simulink library "AEMS_Standard_Library"  (R2016b)
settings: Solver=ode45  StartTime=0.0  StopTime=10.0  RelTol=1e-3
undefined symbols (not defined in the file or in its folder): BkPY, carto, Cbx_extegr, Cbx_lpegrsys, Cbx_portegr, Cnx_bnk_nr_conf, Cnx_cyl_nr_conf, ConfigManagement, configuration_management, Cxx_dcm_io_tmr_end_xxxx, Cxx_dcm_rt_tmr_end, Cxx_DID_xxxx_IO_max, Cxx_DID_xxxx_IO_min, Cxx_egrhsofs, Cxx_vmaniegi, DEM_DEBOUNCE_FREEZE, DEM_DTR_CTL_INVISIBLE, DEM_DTR_CTL_NORMAL, Dem_DtrId2_XXX, Dem_DtrId3_XXX, Dem_DtrId4_XXX, Dem_DtrId5_XXX, Dem_DtrId6_XXX, Dem_DtrId7_XXX, Dem_DtrId8_XXX, Dem_DtrId9_XXX, Dem_DtrId_XXX, Dem_EnableConditionId2_XXX, Dem_EnableConditionId3_XXX, Dem_EnableConditionId4_XXX, Dem_EnableConditionId5_XXX, Dem_EnableConditionId6_XXX, Dem_EnableConditionId7_XXX, Dem_EnableConditionId8_XXX, Dem_EnableConditionId_XXX, Dem_EventId, Dem_EventId2_XXX, Dem_EventId3_XXX, Dem_EventId4_XXX, Dem_EventId5_XXX, Dem_EventId6_XXX, Dem_EventId7_XXX, Dem_EventId8_XXX, Dem_EventId9_XXX, Dem_EventId_Device_Faulttype, Dem_EventId_XXX, DEM_IUMPR_GENERAL_DENOMINATOR, DEM_OPCYC_IGNITION, Dem_RatioId2_XXX, Dem_RatioId3_XXX, Dem_RatioId4_XXX, Dem_RatioId5_XXX, Dem_RatioId6_XXX, Dem_RatioId7_XXX, Dem_RatioId8_XXX, Dem_RatioId_XXX, Dem_StorageConditionId2_XXX, Dem_StorageConditionId3_XXX, Dem_StorageConditionId4_XXX, Dem_StorageConditionId5_XXX ... (+65)
libraries: AEMS_Standard_Library x477, simulink x2
(part 34 of 39)

== system AEMS_Standard_Library/SUB/AEMS_DEM_SET_EVENT_STS_2D/Dem_SetEventStatus_Call2 ==
  dem_event_status_failed2 : Inport
  trigger_job_1st2 : EnablePort
      settings: AttributesFormatString=<states=%<StatesWhenEnabling>>
  AEMS_DEM_SETEVENTSTATUS2 : AEMS_Standard_Library/SUB/AEMS_DEM_SETEVENTSTATUS  Tag=[LIB]
      settings: AttributesFormatString=%<MaskType>
  EventId_block2 : Constant  Value=Dem_EventId2_XXX  OutDataTypeStr=uint16
  wires:
  EventId_block2/1 -> AEMS_DEM_SETEVENTSTATUS2/1
  dem_event_status_failed2/1 -> AEMS_DEM_SETEVENTSTATUS2/2

== system AEMS_Standard_Library/SUB/AEMS_DEM_SET_EVENT_STS_8D/Dem_SetEventStatus_Call1 ==
  dem_event_status_failed1 : Inport
  trigger_job_1st1 : EnablePort
      settings: AttributesFormatString=<states=%<StatesWhenEnabling>>
  AEMS_DEM_SETEVENTSTATUS1 : AEMS_Standard_Library/SUB/AEMS_DEM_SETEVENTSTATUS  Tag=[LIB]
      settings: AttributesFormatString=%<MaskType>
  EventId_block1 : Constant  Value=Dem_EventId_XXX  OutDataTypeStr=uint16
  wires:
  EventId_block1/1 -> AEMS_DEM_SETEVENTSTATUS1/1
  dem_event_status_failed1/1 -> AEMS_DEM_SETEVENTSTATUS1/2

== system AEMS_Standard_Library/SUB/AEMS_DEM_SET_EVENT_STS_8D/Dem_SetEventStatus_Call2 ==
  dem_event_status_failed2 : Inport
  trigger_job_1st2 : EnablePort
      settings: AttributesFormatString=<states=%<StatesWhenEnabling>>
  AEMS_DEM_SETEVENTSTATUS2 : AEMS_Standard_Library/SUB/AEMS_DEM_SETEVENTSTATUS  Tag=[LIB]
      settings: AttributesFormatString=%<MaskType>
  EventId_block2 : Constant  Value=Dem_EventId2_XXX  OutDataTypeStr=uint16
  wires:
  dem_event_status_failed2/1 -> AEMS_DEM_SETEVENTSTATUS2/2
  EventId_block2/1 -> AEMS_DEM_SETEVENTSTATUS2/1

== system AEMS_Standard_Library/SUB/AEMS_DEM_SET_EVENT_STS_8D/Dem_SetEventStatus_Call3 ==
  dem_event_status_failed3 : Inport
  trigger_job_1st3 : EnablePort
      settings: AttributesFormatString=<states=%<StatesWhenEnabling>>
  AEMS_DEM_SETEVENTSTATUS3 : AEMS_Standard_Library/SUB/AEMS_DEM_SETEVENTSTATUS  Tag=[LIB]
      settings: AttributesFormatString=%<MaskType>
  EventId_block3 : Constant  Value=Dem_EventId3_XXX  OutDataTypeStr=uint16
  wires:
  EventId_block3/1 -> AEMS_DEM_SETEVENTSTATUS3/1
  dem_event_status_failed3/1 -> AEMS_DEM_SETEVENTSTATUS3/2

== system AEMS_Standard_Library/SUB/AEMS_DEM_SET_EVENT_STS_8D/Dem_SetEventStatus_Call4 ==
  dem_event_status_failed4 : Inport
  trigger_job_1st4 : EnablePort
      settings: AttributesFormatString=<states=%<StatesWhenEnabling>>
  AEMS_DEM_SETEVENTSTATUS4 : AEMS_Standard_Library/SUB/AEMS_DEM_SETEVENTSTATUS  Tag=[LIB]
      settings: AttributesFormatString=%<MaskType>
  EventId_block4 : Constant  Value=Dem_EventId4_XXX  OutDataTypeStr=uint16
  wires:
  EventId_block4/1 -> AEMS_DEM_SETEVENTSTATUS4/1
  dem_event_status_failed4/1 -> AEMS_DEM_SETEVENTSTATUS4/2

== system AEMS_Standard_Library/SUB/AEMS_DEM_SET_EVENT_STS_8D/Dem_SetEventStatus_Call5 ==
  dem_event_status_failed5 : Inport
  trigger_job_1st5 : EnablePort
      settings: AttributesFormatString=<states=%<StatesWhenEnabling>>
  AEMS_DEM_SETEVENTSTATUS5 : AEMS_Standard_Library/SUB/AEMS_DEM_SETEVENTSTATUS  Tag=[LIB]
      settings: AttributesFormatString=%<MaskType>
  EventId_block5 : Constant  Value=Dem_EventId5_XXX  OutDataTypeStr=uint16
  wires:
  dem_event_status_failed5/1 -> AEMS_DEM_SETEVENTSTATUS5/2
  EventId_block5/1 -> AEMS_DEM_SETEVENTSTATUS5/1

== system AEMS_Standard_Library/SUB/AEMS_DEM_SET_EVENT_STS_8D/Dem_SetEventStatus_Call6 ==
  dem_event_status_failed6 : Inport
  trigger_job_1st6 : EnablePort
      settings: AttributesFormatString=<states=%<StatesWhenEnabling>>
  AEMS_DEM_SETEVENTSTATUS6 : AEMS_Standard_Library/SUB/AEMS_DEM_SETEVENTSTATUS  Tag=[LIB]
      settings: AttributesFormatString=%<MaskType>
  EventId_block6 : Constant  Value=Dem_EventId6_XXX  OutDataTypeStr=uint16
  wires:
  EventId_block6/1 -> AEMS_DEM_SETEVENTSTATUS6/1
  dem_event_status_failed6/1 -> AEMS_DEM_SETEVENTSTATUS6/2

== system AEMS_Standard_Library/SUB/AEMS_DEM_SET_EVENT_STS_8D/Dem_SetEventStatus_Call7 ==
  dem_event_status_failed7 : Inport
  trigger_job_1st7 : EnablePort
      settings: AttributesFormatString=<states=%<StatesWhenEnabling>>
  AEMS_DEM_SETEVENTSTATUS7 : AEMS_Standard_Library/SUB/AEMS_DEM_SETEVENTSTATUS  Tag=[LIB]
      settings: AttributesFormatString=%<MaskType>
  EventId_block7 : Constant  Value=Dem_EventId7_XXX  OutDataTypeStr=uint16
  wires:
  dem_event_status_failed7/1 -> AEMS_DEM_SETEVENTSTATUS7/2
  EventId_block7/1 -> AEMS_DEM_SETEVENTSTATUS7/1

== system AEMS_Standard_Library/SUB/AEMS_DEM_SET_EVENT_STS_8D/Dem_SetEventStatus_Call8 ==
  dem_event_status_failed8 : Inport
  trigger_job_1st8 : EnablePort
      settings: AttributesFormatString=<states=%<StatesWhenEnabling>>
  AEMS_DEM_SETEVENTSTATUS8 : AEMS_Standard_Library/SUB/AEMS_DEM_SETEVENTSTATUS  Tag=[LIB]
      settings: AttributesFormatString=%<MaskType>
  EventId_block8 : Constant  Value=Dem_EventId8_XXX  OutDataTypeStr=uint16
  wires:
  dem_event_status_failed8/1 -> AEMS_DEM_SETEVENTSTATUS8/2
  EventId_block8/1 -> AEMS_DEM_SETEVENTSTATUS8/1

== system AEMS_Standard_Library/SUB/AEMS_DEM_SET_EVENT_STS_9D/Dem_SetEventStatus_Call0 ==
  dem_event_status_failed0 : Inport
      settings: AttributesFormatString=<tsample=%<SampleTime>>
  trigger_job_1st0 : EnablePort
      settings: AttributesFormatString=<states=%<StatesWhenEnabling>>
  AEMS_DEM_SETEVENTSTATUS : AEMS_Standard_Library/SUB/AEMS_DEM_SETEVENTSTATUS  Tag=[LIB]
      settings: AttributesFormatString=%<MaskType>
  EventId_block0 : Constant  Value=Dem_EventId_XXX  OutDataTypeStr=uint16
  wires:
  dem_event_status_failed0/1 -> AEMS_DEM_SETEVENTSTATUS/2
  EventId_block0/1 -> AEMS_DEM_SETEVENTSTATUS/1

== system AEMS_Standard_Library/SUB/AEMS_DEM_SET_EVENT_STS_9D/Dem_SetEventStatus_Call1 ==
  dem_event_status_failed1 : Inport
      settings: AttributesFormatString=<tsample=%<SampleTime>>
  trigger_job_1st1 : EnablePort
      settings: AttributesFormatString=<states=%<StatesWhenEnabling>>
  AEMS_DEM_SETEVENTSTATUS : AEMS_Standard_Library/SUB/AEMS_DEM_SETEVENTSTATUS  Tag=[LIB]
      settings: AttributesFormatString=%<MaskType>
  EventId_block1 : Constant  Value=Dem_EventId2_XXX  OutDataTypeStr=uint16
  wires:
  dem_event_status_failed1/1 -> AEMS_DEM_SETEVENTSTATUS/2
  EventId_block1/1 -> AEMS_DEM_SETEVENTSTATUS/1

== system AEMS_Standard_Library/SUB/AEMS_DEM_SET_EVENT_STS_9D/Dem_SetEventStatus_Call2 ==
  dem_event_status_failed2 : Inport
      settings: AttributesFormatString=<tsample=%<SampleTime>>
  trigger_job_1st2 : EnablePort
      settings: AttributesFormatString=<states=%<StatesWhenEnabling>>
  AEMS_DEM_SETEVENTSTATUS : AEMS_Standard_Library/SUB/AEMS_DEM_SETEVENTSTATUS  Tag=[LIB]
      settings: AttributesFormatString=%<MaskType>
  EventId_block2 : Constant  Value=Dem_EventId3_XXX  OutDataTypeStr=uint16
  wires:
  EventId_block2/1 -> AEMS_DEM_SETEVENTSTATUS/1
  dem_event_status_failed2/1 -> AEMS_DEM_SETEVENTSTATUS/2

== system AEMS_Standard_Library/SUB/AEMS_DEM_SET_EVENT_STS_9D/Dem_SetEventStatus_Call3 ==
  dem_event_status_failed3 : Inport
      settings: AttributesFormatString=<tsample=%<SampleTime>>
  trigger_job_1st3 : EnablePort
      settings: AttributesFormatString=<states=%<StatesWhenEnabling>>
  AEMS_DEM_SETEVENTSTATUS : AEMS_Standard_Library/SUB/AEMS_DEM_SETEVENTSTATUS  Tag=[LIB]
      settings: AttributesFormatString=%<MaskType>
  EventId_block3 : Constant  Value=Dem_EventId4_XXX  OutDataTypeStr=uint16
  wires:
  dem_event_status_failed3/1 -> AEMS_DEM_SETEVENTSTATUS/2
  EventId_block3/1 -> AEMS_DEM_SETEVENTSTATUS/1

== system AEMS_Standard_Library/SUB/AEMS_DEM_SET_EVENT_STS_9D/Dem_SetEventStatus_Call4 ==
  dem_event_status_failed4 : Inport
      settings: AttributesFormatString=<tsample=%<SampleTime>>
  trigger_job_1st4 : EnablePort
      settings: AttributesFormatString=<states=%<StatesWhenEnabling>>
  AEMS_DEM_SETEVENTSTATUS : AEMS_Standard_Library/SUB/AEMS_DEM_SETEVENTSTATUS  Tag=[LIB]
      settings: AttributesFormatString=%<MaskType>
  EventId_block4 : Constant  Value=Dem_EventId5_XXX  OutDataTypeStr=uint16
  wires:
  dem_event_status_failed4/1 -> AEMS_DEM_SETEVENTSTATUS/2
  EventId_block4/1 -> AEMS_DEM_SETEVENTSTATUS/1

== system AEMS_Standard_Library/SUB/AEMS_DEM_SET_EVENT_STS_9D/Dem_SetEventStatus_Call5 ==
  dem_event_status_failed5 : Inport
      settings: AttributesFormatString=<tsample=%<SampleTime>>
  trigger_job_1st5 : EnablePort
      settings: AttributesFormatString=<states=%<StatesWhenEnabling>>
  AEMS_DEM_SETEVENTSTATUS : AEMS_Standard_Library/SUB/AEMS_DEM_SETEVENTSTATUS  Tag=[LIB]
      settings: AttributesFormatString=%<MaskType>
  EventId_block5 : Constant  Value=Dem_EventId6_XXX  OutDataTypeStr=uint16
  wires:
  EventId_block5/1 -> AEMS_DEM_SETEVENTSTATUS/1
  dem_event_status_failed5/1 -> AEMS_DEM_SETEVENTSTATUS/2

== system AEMS_Standard_Library/SUB/AEMS_DEM_SET_EVENT_STS_9D/Dem_SetEventStatus_Call6 ==
  dem_event_status_failed6 : Inport
      settings: AttributesFormatString=<tsample=%<SampleTime>>
  trigger_job_1st6 : EnablePort
      settings: AttributesFormatString=<states=%<StatesWhenEnabling>>
  AEMS_DEM_SETEVENTSTATUS : AEMS_Standard_Library/SUB/AEMS_DEM_SETEVENTSTATUS  Tag=[LIB]
      settings: AttributesFormatString=%<MaskType>
  EventId_block6 : Constant  Value=Dem_EventId7_XXX  OutDataTypeStr=uint16
  wires:
  dem_event_status_failed6/1 -> AEMS_DEM_SETEVENTSTATUS/2
  EventId_block6/1 -> AEMS_DEM_SETEVENTSTATUS/1

== system AEMS_Standard_Library/SUB/AEMS_DEM_SET_EVENT_STS_9D/Dem_SetEventStatus_Call7 ==
  dem_event_status_failed7 : Inport
      settings: AttributesFormatString=<tsample=%<SampleTime>>
  trigger_job_1st7 : EnablePort
      settings: AttributesFormatString=<states=%<StatesWhenEnabling>>
  AEMS_DEM_SETEVENTSTATUS : AEMS_Standard_Library/SUB/AEMS_DEM_SETEVENTSTATUS  Tag=[LIB]
      settings: AttributesFormatString=%<MaskType>
  EventId_block7 : Constant  Value=Dem_EventId8_XXX  OutDataTypeStr=uint16
  wires:
  EventId_block7/1 -> AEMS_DEM_SETEVENTSTATUS/1
  dem_event_status_failed7/1 -> AEMS_DEM_SETEVENTSTATUS/2

== system AEMS_Standard_Library/SUB/AEMS_DEM_SET_EVENT_STS_9D/Dem_SetEventStatus_Call8 ==
  dem_event_status_failed8 : Inport
      settings: AttributesFormatString=<tsample=%<SampleTime>>
  trigger_job_1st8 : EnablePort
      settings: AttributesFormatString=<states=%<StatesWhenEnabling>>
  AEMS_DEM_SETEVENTSTATUS : AEMS_Standard_Library/SUB/AEMS_DEM_SETEVENTSTATUS  Tag=[LIB]
      settings: AttributesFormatString=%<MaskType>
  EventId_block8 : Constant  Value=Dem_EventId9_XXX  OutDataTypeStr=uint16
  wires:
  EventId_block8/1 -> AEMS_DEM_SETEVENTSTATUS/1
  dem_event_status_failed8/1 -> AEMS_DEM_SETEVENTSTATUS/2

== system AEMS_Standard_Library/SUB/AEMS_DEM_TIMEBASEDDEBOUNCE/Dem_SetEventStatus_Call ==
  event_status : Inport
  call_seteventstatus : EnablePort
      settings: AttributesFormatString=<states=%<StatesWhenEnabling>>
  AEMS_DEM_SETEVENTSTATUS : AEMS_Standard_Library/SUB/AEMS_DEM_SETEVENTSTATUS  Tag=[LIB]
      settings: AttributesFormatString=%<MaskType>
  EventId_block : Constant  Value=Dem_EventId  OutDataTypeStr=uint16
  wires:
  event_status/1 -> AEMS_DEM_SETEVENTSTATUS/2
  EventId_block/1 -> AEMS_DEM_SETEVENTSTATUS/1

== system AEMS_Standard_Library/SUB/AEMS_DEM_TIMEBASEDDEBOUNCE/Subsystem_Timer_Debounce_Call ==
  conditionfulfilled : Inport  OutDataTypeStr=boolean
  prefailed : Inport  Port=2  OutDataTypeStr=boolean
  prepassed : Inport  Port=3  OutDataTypeStr=boolean
  behavior : Inport  Port=4  OutDataTypeStr=uint8
  failedthreshold : Inport  Port=5  OutDataTypeStr=single
  passedthreshold : Inport  Port=6  OutDataTypeStr=single
  reseteventdebounce : Inport  Port=7  OutDataTypeStr=boolean
  AEMS_EDGE_RISING : AEMS_Standard_Library/EDGE/AEMS_EDGE_RISING  Tag=[LIB]  init=false
      settings: AttributesFormatString=|
      | %<MaskType>
      | Initial Value : %<init>
  AEMS_EDGE_RISING1 : AEMS_Standard_Library/EDGE/AEMS_EDGE_RISING  Tag=[LIB]  init=false
      settings: AttributesFormatString=|
      | %<MaskType>
      | Initial Value : %<init>
  AEMS_TIMER_H : AEMS_Standard_Library/TIMER/AEMS_TIMER_H  Tag=[LIB]  sample_time=0.01
      settings: AttributesFormatString=%<MaskType>
  AEMS_TIMER_H1 : AEMS_Standard_Library/TIMER/AEMS_TIMER_H  Tag=[LIB]  sample_time=0.01
      settings: AttributesFormatString=%<MaskType>
  DemTimeBypassFailure : Constant  Value=DemTimeBypassFailure
  Logical Operator : Logic  Operator=OR  OutDataTypeStr=boolean
  Logical Operator1 : Logic  OutDataTypeStr=boolean
  Logical Operator3 : Logic  Operator=NOT  OutDataTypeStr=boolean
  LogicalOperator11 : Logic  Operator=NOT  Inputs=1  OutDataTypeStr=boolean
  LogicalOperator2 : Logic  Operator=OR  Inputs=3  OutDataTypeStr=boolean
  LogicalOperator3 : Logic  Operator=OR  OutDataTypeStr=boolean
  LogicalOperator4 : Logic  Operator=NOT  Inputs=1  OutDataTypeStr=boolean
  LogicalOperator{5..7,9} (4 alike) : Logic  OutDataTypeStr=boolean
  LogicalOperator8 : Logic  Operator=OR  Inputs=3  OutDataTypeStr=boolean
  RelationalOperator : RelationalOperator  Operator===  OutDataTypeStr=boolean  RndMeth=Nearest  InputSameDT=on
  Saturation : Saturate  UpperLimit=3600  LowerLimit=0.001
      settings: AttributesFormatString=<limits=%<UpperLimit>/%<LowerLimit>>
  Saturation2 : Saturate  UpperLimit=3600  LowerLimit=0.001
      settings: AttributesFormatString=<limits=%<UpperLimit>/%<LowerLimit>>
  Switch7 : Switch  Threshold=0.5  SaturateOnIntegerOverflow=on  InputSameDT=on
  behavior_case : Constant  OutDataTypeStr=uint8
  status_failed : Constant  OutDataTypeStr=uint8
  status_passed : Constant  Value=0  OutDataTypeStr=uint8
  debouncevalue_for_failed : Outport
  debouncevalue_for_passed : Outport  Port=2
  failed : Outport  Port=3
  passed : Outport  Port=4
  call_seteventstatus : Outport  Port=5
  eventstatus : Outport  Port=6
  wires:
  Logical Operator3/1 -> Logical Operator1/1
  AEMS_TIMER_H/1 -> Logical Operator1/2  "passed"
  Logical Operator1/1 -> passed/1, AEMS_EDGE_RISING1/1
  Logical Operator/1 -> Logical Operator3/1, AEMS_EDGE_RISING/1, Switch7/2, failed/1
  DemTimeBypassFailure/1 -> Logical Operator/1
  AEMS_TIMER_H1/1 -> Logical Operator/2
  LogicalOperator7/1 -> AEMS_TIMER_H/1, LogicalOperator8/3, LogicalOperator11/1
  prepassed/1 -> LogicalOperator7/2
  LogicalOperator5/1 -> AEMS_TIMER_H1/1, LogicalOperator4/1
  conditionfulfilled/1 -> LogicalOperator7/1, LogicalOperator5/2  "conditionfulfilled"
  AEMS_TIMER_H1/2 -> debouncevalue_for_failed/1  "debouncevalue_for_failed"
  AEMS_TIMER_H/2 -> debouncevalue_for_passed/1  "debouncevalue_for_passed"
  LogicalOperator9/1 -> LogicalOperator2/2
  LogicalOperator11/1 -> LogicalOperator9/1
  LogicalOperator2/1 -> AEMS_TIMER_H/2
  LogicalOperator4/1 -> LogicalOperator6/1
  LogicalOperator8/1 -> AEMS_TIMER_H1/2
  LogicalOperator6/1 -> LogicalOperator8/1
  Saturation/1 -> AEMS_TIMER_H1/3
  behavior/1 -> RelationalOperator/1
  failedthreshold/1 -> Saturation/1
  prefailed/1 -> LogicalOperator2/3, LogicalOperator5/1
  passedthreshold/1 -> Saturation2/1
  behavior_case/1 -> RelationalOperator/2
  RelationalOperator/1 -> LogicalOperator6/2, LogicalOperator9/2
  reseteventdebounce/1 -> LogicalOperator8/2, LogicalOperator2/1
  Saturation2/1 -> AEMS_TIMER_H/3
  status_failed/1 -> Switch7/1
  status_passed/1 -> Switch7/3
  Switch7/1 -> eventstatus/1  "eventstatus"
  AEMS_EDGE_RISING/1 -> LogicalOperator3/1
  AEMS_EDGE_RISING1/1 -> LogicalOperator3/2
  LogicalOperator3/1 -> call_seteventstatus/1  "call_seteventstatus"

== system AEMS_Standard_Library/SUB/AEMS_DEM_TIME_BASED_DEBOUNCE_1D/AEMS_DEM_TIME_BASED_DEBOUNCE_CALL ==
  conditionfulfilled : Inport
  prefailed : Inport  Port=2
  prepassed : Inport  Port=3
  reseteventdebounce : Inport  Port=4
  DemDebounceBehavior : Inport  Port=5
  DemCounterFailedThreshold : Inport  Port=6
  DemCounterPassedThreshold : Inport  Port=7
  Enable : EnablePort
      settings: AttributesFormatString=StatesWhenEnabling = %<StatesWhenEnabling>
  AEMS_DEM_TIMEBASEDDEBOUNCE : AEMS_Standard_Library/SUB/AEMS_DEM_TIMEBASEDDEBOUNCE  Tag=[LIB]  eventid=Dem_EventId_Device_Faulttype  sampletime=0.01
      settings: AttributesFormatString=|
      | %<MaskType>
      | EventId: %<eventid>
      | Sample time: %<sampletime>
  debouncevalue_for_failed : Outport
      settings: AttributesFormatString=<initial=%<InitialOutput>>\n<whendisabled=%<OutputWhenDisabled>>
  debouncevalue_for_passed : Outport  Port=2
      settings: AttributesFormatString=<initial=%<InitialOutput>>\n<whendisabled=%<OutputWhenDisabled>>
  failed : Outport  Port=3
      settings: AttributesFormatString=<initial=%<InitialOutput>>\n<whendisabled=%<OutputWhenDisabled>>
  passed : Outport  Port=4
      settings: AttributesFormatString=<initial=%<InitialOutput>>\n<whendisabled=%<OutputWhenDisabled>>
  wires:
  DemCounterPassedThreshold/1 -> AEMS_DEM_TIMEBASEDDEBOUNCE/6
  DemDebounceBehavior/1 -> AEMS_DEM_TIMEBASEDDEBOUNCE/4
  conditionfulfilled/1 -> AEMS_DEM_TIMEBASEDDEBOUNCE/1
  prepassed/1 -> AEMS_DEM_TIMEBASEDDEBOUNCE/3
  reseteventdebounce/1 -> AEMS_DEM_TIMEBASEDDEBOUNCE/7
  prefailed/1 -> AEMS_DEM_TIMEBASEDDEBOUNCE/2
  DemCounterFailedThreshold/1 -> AEMS_DEM_TIMEBASEDDEBOUNCE/5
  AEMS_DEM_TIMEBASEDDEBOUNCE/1 -> debouncevalue_for_failed/1
  AEMS_DEM_TIMEBASEDDEBOUNCE/2 -> debouncevalue_for_passed/1
  AEMS_DEM_TIMEBASEDDEBOUNCE/3 -> failed/1
  AEMS_DEM_TIMEBASEDDEBOUNCE/4 -> passed/1

== system AEMS_Standard_Library/SUB/AEMS_DEM_TIME_BASED_DEBOUNCE_2D/AEMS_DEM_TIME_BASED_DEBOUNCE_CALL1 ==
  conditionfulfilled : Inport
  prefailed : Inport  Port=2
  prepassed : Inport  Port=3
  reseteventdebounce : Inport  Port=4
  DemDebounceBehavior : Inport  Port=5
  DemCounterFailedThreshold : Inport  Port=6
  DemCounterPassedThreshold : Inport  Port=7
  Enable : EnablePort
  AEMS_DEM_TIMEBASEDDEBOUNCE : AEMS_Standard_Library/SUB/AEMS_DEM_TIMEBASEDDEBOUNCE  Tag=[LIB]  eventid=Dem_EventId_Device_Faulttype  sampletime=0.01
      settings: AttributesFormatString=|
      | %<MaskType>
      | EventId: %<eventid>
      | Sample time: %<sampletime>
  debouncevalue_for_failed : Outport
  debouncevalue_for_passed : Outport  Port=2
  failed : Outport  Port=3
  passed : Outport  Port=4
  wires:
  AEMS_DEM_TIMEBASEDDEBOUNCE/4 -> passed/1
  AEMS_DEM_TIMEBASEDDEBOUNCE/3 -> failed/1
  AEMS_DEM_TIMEBASEDDEBOUNCE/2 -> debouncevalue_for_passed/1
  AEMS_DEM_TIMEBASEDDEBOUNCE/1 -> debouncevalue_for_failed/1
  DemCounterFailedThreshold/1 -> AEMS_DEM_TIMEBASEDDEBOUNCE/5
  prefailed/1 -> AEMS_DEM_TIMEBASEDDEBOUNCE/2
  reseteventdebounce/1 -> AEMS_DEM_TIMEBASEDDEBOUNCE/7
  prepassed/1 -> AEMS_DEM_TIMEBASEDDEBOUNCE/3
  conditionfulfilled/1 -> AEMS_DEM_TIMEBASEDDEBOUNCE/1
  DemDebounceBehavior/1 -> AEMS_DEM_TIMEBASEDDEBOUNCE/4
  DemCounterPassedThreshold/1 -> AEMS_DEM_TIMEBASEDDEBOUNCE/6

== system AEMS_Standard_Library/SUB/AEMS_DEM_TIME_BASED_DEBOUNCE_2D/AEMS_DEM_TIME_BASED_DEBOUNCE_CALL2 ==
  conditionfulfilled : Inport
  prefailed : Inport  Port=2
  prepassed : Inport  Port=3
  reseteventdebounce : Inport  Port=4
  DemDebounceBehavior : Inport  Port=5
  DemCounterFailedThreshold : Inport  Port=6
  DemCounterPassedThreshold : Inport  Port=7
  Enable : EnablePort
  AEMS_DEM_TIMEBASEDDEBOUNCE : AEMS_Standard_Library/SUB/AEMS_DEM_TIMEBASEDDEBOUNCE  Tag=[LIB]  eventid=Dem_EventId_Device2_Faulttype  sampletime=0.01
      settings: AttributesFormatString=|
      | %<MaskType>
      | EventId: %<eventid>
      | Sample time: %<sampletime>
  debouncevalue_for_failed : Outport
  debouncevalue_for_passed : Outport  Port=2
  failed : Outport  Port=3
  passed : Outport  Port=4
  wires:
  DemCounterPassedThreshold/1 -> AEMS_DEM_TIMEBASEDDEBOUNCE/6
  DemDebounceBehavior/1 -> AEMS_DEM_TIMEBASEDDEBOUNCE/4
  conditionfulfilled/1 -> AEMS_DEM_TIMEBASEDDEBOUNCE/1
  prepassed/1 -> AEMS_DEM_TIMEBASEDDEBOUNCE/3
  reseteventdebounce/1 -> AEMS_DEM_TIMEBASEDDEBOUNCE/7
  prefailed/1 -> AEMS_DEM_TIMEBASEDDEBOUNCE/2
  DemCounterFailedThreshold/1 -> AEMS_DEM_TIMEBASEDDEBOUNCE/5
  AEMS_DEM_TIMEBASEDDEBOUNCE/1 -> debouncevalue_for_failed/1
  AEMS_DEM_TIMEBASEDDEBOUNCE/2 -> debouncevalue_for_passed/1
  AEMS_DEM_TIMEBASEDDEBOUNCE/3 -> failed/1
  AEMS_DEM_TIMEBASEDDEBOUNCE/4 -> passed/1

== system AEMS_Standard_Library/SUB/AEMS_DEM_TIME_BASED_DEBOUNCE_3D/AEMS_DEM_TIME_BASED_DEBOUNCE_CALL1 ==
  conditionfulfilled : Inport
  prefailed : Inport  Port=2
  prepassed : Inport  Port=3
  reseteventdebounce : Inport  Port=4
  DemDebounceBehavior : Inport  Port=5
  DemCounterFailedThreshold : Inport  Port=6
  DemCounterPassedThreshold : Inport  Port=7
  Enable : EnablePort
  AEMS_DEM_TIMEBASEDDEBOUNCE : AEMS_Standard_Library/SUB/AEMS_DEM_TIMEBASEDDEBOUNCE  Tag=[LIB]  eventid=Dem_EventId_Device_Faulttype  sampletime=0.1
      settings: AttributesFormatString=|
      | %<MaskType>
      | EventId: %<eventid>
      | Sample time: %<sampletime>
  debouncevalue_for_failed : Outport
  debouncevalue_for_passed : Outport  Port=2
  failed : Outport  Port=3
  passed : Outport  Port=4
  wires:
  AEMS_DEM_TIMEBASEDDEBOUNCE/4 -> passed/1
  AEMS_DEM_TIMEBASEDDEBOUNCE/3 -> failed/1
  AEMS_DEM_TIMEBASEDDEBOUNCE/2 -> debouncevalue_for_passed/1
  AEMS_DEM_TIMEBASEDDEBOUNCE/1 -> debouncevalue_for_failed/1
  DemCounterFailedThreshold/1 -> AEMS_DEM_TIMEBASEDDEBOUNCE/5
  prefailed/1 -> AEMS_DEM_TIMEBASEDDEBOUNCE/2
  reseteventdebounce/1 -> AEMS_DEM_TIMEBASEDDEBOUNCE/7
  prepassed/1 -> AEMS_DEM_TIMEBASEDDEBOUNCE/3
  conditionfulfilled/1 -> AEMS_DEM_TIMEBASEDDEBOUNCE/1
  DemDebounceBehavior/1 -> AEMS_DEM_TIMEBASEDDEBOUNCE/4
  DemCounterPassedThreshold/1 -> AEMS_DEM_TIMEBASEDDEBOUNCE/6

== system AEMS_Standard_Library/SUB/AEMS_DEM_TIME_BASED_DEBOUNCE_3D/AEMS_DEM_TIME_BASED_DEBOUNCE_CALL2 ==
  conditionfulfilled : Inport
  prefailed : Inport  Port=2
  prepassed : Inport  Port=3
  reseteventdebounce : Inport  Port=4
  DemDebounceBehavior : Inport  Port=5
  DemCounterFailedThreshold : Inport  Port=6
  DemCounterPassedThreshold : Inport  Port=7
  Enable : EnablePort
  AEMS_DEM_TIMEBASEDDEBOUNCE : AEMS_Standard_Library/SUB/AEMS_DEM_TIMEBASEDDEBOUNCE  Tag=[LIB]  eventid=Dem_EventId_Device2_Faulttype  sampletime=0.1
      settings: AttributesFormatString=|
      | %<MaskType>
      | EventId: %<eventid>
      | Sample time: %<sampletime>
  debouncevalue_for_failed : Outport
  debouncevalue_for_passed : Outport  Port=2
  failed : Outport  Port=3
  passed : Outport  Port=4
  wires:
  DemCounterPassedThreshold/1 -> AEMS_DEM_TIMEBASEDDEBOUNCE/6
  DemDebounceBehavior/1 -> AEMS_DEM_TIMEBASEDDEBOUNCE/4
  conditionfulfilled/1 -> AEMS_DEM_TIMEBASEDDEBOUNCE/1
  prepassed/1 -> AEMS_DEM_TIMEBASEDDEBOUNCE/3
  reseteventdebounce/1 -> AEMS_DEM_TIMEBASEDDEBOUNCE/7
  prefailed/1 -> AEMS_DEM_TIMEBASEDDEBOUNCE/2
  DemCounterFailedThreshold/1 -> AEMS_DEM_TIMEBASEDDEBOUNCE/5
  AEMS_DEM_TIMEBASEDDEBOUNCE/1 -> debouncevalue_for_failed/1
  AEMS_DEM_TIMEBASEDDEBOUNCE/2 -> debouncevalue_for_passed/1
  AEMS_DEM_TIMEBASEDDEBOUNCE/3 -> failed/1
  AEMS_DEM_TIMEBASEDDEBOUNCE/4 -> passed/1

== system AEMS_Standard_Library/SUB/AEMS_DEM_TIME_BASED_DEBOUNCE_3D/AEMS_DEM_TIME_BASED_DEBOUNCE_CALL3 ==
  conditionfulfilled : Inport
  prefailed : Inport  Port=2
  prepassed : Inport  Port=3
  reseteventdebounce : Inport  Port=4
  DemDebounceBehavior : Inport  Port=5
  DemCounterFailedThreshold : Inport  Port=6
  DemCounterPassedThreshold : Inport  Port=7
  Enable : EnablePort
  AEMS_DEM_TIMEBASEDDEBOUNCE : AEMS_Standard_Library/SUB/AEMS_DEM_TIMEBASEDDEBOUNCE  Tag=[LIB]  eventid=Dem_EventId_Device3_Faulttype  sampletime=0.1
      settings: AttributesFormatString=|
      | %<MaskType>
      | EventId: %<eventid>
      | Sample time: %<sampletime>
  debouncevalue_for_failed : Outport
  debouncevalue_for_passed : Outport  Port=2
  failed : Outport  Port=3
  passed : Outport  Port=4
  wires:
  DemCounterPassedThreshold/1 -> AEMS_DEM_TIMEBASEDDEBOUNCE/6
  DemDebounceBehavior/1 -> AEMS_DEM_TIMEBASEDDEBOUNCE/4
  conditionfulfilled/1 -> AEMS_DEM_TIMEBASEDDEBOUNCE/1
  prepassed/1 -> AEMS_DEM_TIMEBASEDDEBOUNCE/3
  reseteventdebounce/1 -> AEMS_DEM_TIMEBASEDDEBOUNCE/7
  prefailed/1 -> AEMS_DEM_TIMEBASEDDEBOUNCE/2
  DemCounterFailedThreshold/1 -> AEMS_DEM_TIMEBASEDDEBOUNCE/5
  AEMS_DEM_TIMEBASEDDEBOUNCE/1 -> debouncevalue_for_failed/1
  AEMS_DEM_TIMEBASEDDEBOUNCE/2 -> debouncevalue_for_passed/1
  AEMS_DEM_TIMEBASEDDEBOUNCE/3 -> failed/1
  AEMS_DEM_TIMEBASEDDEBOUNCE/4 -> passed/1

== system AEMS_Standard_Library/SUB/AEMS_DEM_TIME_BASED_DEBOUNCE_4D/AEMS_DEM_TIME_BASED_DEBOUNCE_CALL1 ==
  conditionfulfilled : Inport
  prefailed : Inport  Port=2
  prepassed : Inport  Port=3
  reseteventdebounce : Inport  Port=4
  DemDebounceBehavior : Inport  Port=5
  DemCounterFailedThreshold : Inport  Port=6
  DemCounterPassedThreshold : Inport  Port=7
  Enable : EnablePort
  AEMS_DEM_TIMEBASEDDEBOUNCE : AEMS_Standard_Library/SUB/AEMS_DEM_TIMEBASEDDEBOUNCE  Tag=[LIB]  eventid=Dem_EventId_Device_Faulttype  sampletime=0.01
      settings: AttributesFormatString=|
      | %<MaskType>
      | EventId: %<eventid>
      | Sample time: %<sampletime>
  debouncevalue_for_failed : Outport
  debouncevalue_for_passed : Outport  Port=2
  failed : Outport  Port=3
  passed : Outport  Port=4
  wires:
  AEMS_DEM_TIMEBASEDDEBOUNCE/4 -> passed/1
  AEMS_DEM_TIMEBASEDDEBOUNCE/3 -> failed/1
  AEMS_DEM_TIMEBASEDDEBOUNCE/2 -> debouncevalue_for_passed/1
  AEMS_DEM_TIMEBASEDDEBOUNCE/1 -> debouncevalue_for_failed/1
  DemCounterFailedThreshold/1 -> AEMS_DEM_TIMEBASEDDEBOUNCE/5
  prefailed/1 -> AEMS_DEM_TIMEBASEDDEBOUNCE/2
  reseteventdebounce/1 -> AEMS_DEM_TIMEBASEDDEBOUNCE/7
  prepassed/1 -> AEMS_DEM_TIMEBASEDDEBOUNCE/3
  conditionfulfilled/1 -> AEMS_DEM_TIMEBASEDDEBOUNCE/1
  DemDebounceBehavior/1 -> AEMS_DEM_TIMEBASEDDEBOUNCE/4
  DemCounterPassedThreshold/1 -> AEMS_DEM_TIMEBASEDDEBOUNCE/6

== system AEMS_Standard_Library/SUB/AEMS_DEM_TIME_BASED_DEBOUNCE_4D/AEMS_DEM_TIME_BASED_DEBOUNCE_CALL2 ==
  conditionfulfilled : Inport
  prefailed : Inport  Port=2
  prepassed : Inport  Port=3
  reseteventdebounce : Inport  Port=4
  DemDebounceBehavior : Inport  Port=5
  DemCounterFailedThreshold : Inport  Port=6
  DemCounterPassedThreshold : Inport  Port=7
  Enable : EnablePort
  AEMS_DEM_TIMEBASEDDEBOUNCE : AEMS_Standard_Library/SUB/AEMS_DEM_TIMEBASEDDEBOUNCE  Tag=[LIB]  eventid=Dem_EventId_Device2_Faulttype  sampletime=0.01
      settings: AttributesFormatString=|
      | %<MaskType>
      | EventId: %<eventid>
      | Sample time: %<sampletime>
  debouncevalue_for_failed : Outport
  debouncevalue_for_passed : Outport  Port=2
  failed : Outport  Port=3
  passed : Outport  Port=4
  wires:
  DemCounterPassedThreshold/1 -> AEMS_DEM_TIMEBASEDDEBOUNCE/6
  DemDebounceBehavior/1 -> AEMS_DEM_TIMEBASEDDEBOUNCE/4
  conditionfulfilled/1 -> AEMS_DEM_TIMEBASEDDEBOUNCE/1
  prepassed/1 -> AEMS_DEM_TIMEBASEDDEBOUNCE/3
  reseteventdebounce/1 -> AEMS_DEM_TIMEBASEDDEBOUNCE/7
  prefailed/1 -> AEMS_DEM_TIMEBASEDDEBOUNCE/2
  DemCounterFailedThreshold/1 -> AEMS_DEM_TIMEBASEDDEBOUNCE/5
  AEMS_DEM_TIMEBASEDDEBOUNCE/1 -> debouncevalue_for_failed/1
  AEMS_DEM_TIMEBASEDDEBOUNCE/2 -> debouncevalue_for_passed/1
  AEMS_DEM_TIMEBASEDDEBOUNCE/3 -> failed/1
  AEMS_DEM_TIMEBASEDDEBOUNCE/4 -> passed/1

== system AEMS_Standard_Library/SUB/AEMS_DEM_TIME_BASED_DEBOUNCE_4D/AEMS_DEM_TIME_BASED_DEBOUNCE_CALL3 ==
  conditionfulfilled : Inport
  prefailed : Inport  Port=2
  prepassed : Inport  Port=3
  reseteventdebounce : Inport  Port=4
  DemDebounceBehavior : Inport  Port=5
  DemCounterFailedThreshold : Inport  Port=6
  DemCounterPassedThreshold : Inport  Port=7
  Enable : EnablePort
  AEMS_DEM_TIMEBASEDDEBOUNCE : AEMS_Standard_Library/SUB/AEMS_DEM_TIMEBASEDDEBOUNCE  Tag=[LIB]  eventid=Dem_EventId_Device3_Faulttype  sampletime=0.01
      settings: AttributesFormatString=|
      | %<MaskType>
      | EventId: %<eventid>
      | Sample time: %<sampletime>
  debouncevalue_for_failed : Outport
  debouncevalue_for_passed : Outport  Port=2
  failed : Outport  Port=3
  passed : Outport  Port=4
  wires:
  DemCounterPassedThreshold/1 -> AEMS_DEM_TIMEBASEDDEBOUNCE/6
  DemDebounceBehavior/1 -> AEMS_DEM_TIMEBASEDDEBOUNCE/4
  conditionfulfilled/1 -> AEMS_DEM_TIMEBASEDDEBOUNCE/1
  prepassed/1 -> AEMS_DEM_TIMEBASEDDEBOUNCE/3
  reseteventdebounce/1 -> AEMS_DEM_TIMEBASEDDEBOUNCE/7
  prefailed/1 -> AEMS_DEM_TIMEBASEDDEBOUNCE/2
  DemCounterFailedThreshold/1 -> AEMS_DEM_TIMEBASEDDEBOUNCE/5
  AEMS_DEM_TIMEBASEDDEBOUNCE/1 -> debouncevalue_for_failed/1
  AEMS_DEM_TIMEBASEDDEBOUNCE/2 -> debouncevalue_for_passed/1
  AEMS_DEM_TIMEBASEDDEBOUNCE/3 -> failed/1
  AEMS_DEM_TIMEBASEDDEBOUNCE/4 -> passed/1

== system AEMS_Standard_Library/SUB/AEMS_DEM_TIME_BASED_DEBOUNCE_4D/AEMS_DEM_TIME_BASED_DEBOUNCE_CALL4 ==
  conditionfulfilled : Inport
  prefailed : Inport  Port=2
  prepassed : Inport  Port=3
  reseteventdebounce : Inport  Port=4
  DemDebounceBehavior : Inport  Port=5
  DemCounterFailedThreshold : Inport  Port=6
  DemCounterPassedThreshold : Inport  Port=7
  Enable : EnablePort
  AEMS_DEM_TIMEBASEDDEBOUNCE : AEMS_Standard_Library/SUB/AEMS_DEM_TIMEBASEDDEBOUNCE  Tag=[LIB]  eventid=Dem_EventId_Device4_Faulttype  sampletime=0.01
      settings: AttributesFormatString=|
      | %<MaskType>
      | EventId: %<eventid>
      | Sample time: %<sampletime>
  debouncevalue_for_failed : Outport
  debouncevalue_for_passed : Outport  Port=2
  failed : Outport  Port=3
  passed : Outport  Port=4
  wires:
  DemCounterPassedThreshold/1 -> AEMS_DEM_TIMEBASEDDEBOUNCE/6
  DemDebounceBehavior/1 -> AEMS_DEM_TIMEBASEDDEBOUNCE/4
  conditionfulfilled/1 -> AEMS_DEM_TIMEBASEDDEBOUNCE/1
  prepassed/1 -> AEMS_DEM_TIMEBASEDDEBOUNCE/3
  reseteventdebounce/1 -> AEMS_DEM_TIMEBASEDDEBOUNCE/7
  prefailed/1 -> AEMS_DEM_TIMEBASEDDEBOUNCE/2
  DemCounterFailedThreshold/1 -> AEMS_DEM_TIMEBASEDDEBOUNCE/5
  AEMS_DEM_TIMEBASEDDEBOUNCE/1 -> debouncevalue_for_failed/1
  AEMS_DEM_TIMEBASEDDEBOUNCE/2 -> debouncevalue_for_passed/1
  AEMS_DEM_TIMEBASEDDEBOUNCE/3 -> failed/1
  AEMS_DEM_TIMEBASEDDEBOUNCE/4 -> passed/1

== system AEMS_Standard_Library/SUB/AEMS_DEM_TIME_BASED_DEBOUNCE_6D/AEMS_DEM_TIME_BASED_DEBOUNCE_CALL1 ==
  conditionfulfilled : Inport
  prefailed : Inport  Port=2
  prepassed : Inport  Port=3
  reseteventdebounce : Inport  Port=4
  DemDebounceBehavior : Inport  Port=5
  DemCounterFailedThreshold : Inport  Port=6
  DemCounterPassedThreshold : Inport  Port=7
  Enable : EnablePort
  AEMS_DEM_TIMEBASEDDEBOUNCE : AEMS_Standard_Library/SUB/AEMS_DEM_TIMEBASEDDEBOUNCE  Tag=[LIB]  eventid=Dem_EventId_Device_Faulttype  sampletime=0.01
      settings: AttributesFormatString=|
      | %<MaskType>
      | EventId: %<eventid>
      | Sample time: %<sampletime>
  debouncevalue_for_failed : Outport
  debouncevalue_for_passed : Outport  Port=2
  failed : Outport  Port=3
  passed : Outport  Port=4
  wires:
  AEMS_DEM_TIMEBASEDDEBOUNCE/4 -> passed/1
  AEMS_DEM_TIMEBASEDDEBOUNCE/3 -> failed/1
  AEMS_DEM_TIMEBASEDDEBOUNCE/2 -> debouncevalue_for_passed/1
  AEMS_DEM_TIMEBASEDDEBOUNCE/1 -> debouncevalue_for_failed/1
  DemCounterFailedThreshold/1 -> AEMS_DEM_TIMEBASEDDEBOUNCE/5
  prefailed/1 -> AEMS_DEM_TIMEBASEDDEBOUNCE/2
  reseteventdebounce/1 -> AEMS_DEM_TIMEBASEDDEBOUNCE/7
  prepassed/1 -> AEMS_DEM_TIMEBASEDDEBOUNCE/3
  conditionfulfilled/1 -> AEMS_DEM_TIMEBASEDDEBOUNCE/1
  DemDebounceBehavior/1 -> AEMS_DEM_TIMEBASEDDEBOUNCE/4
  DemCounterPassedThreshold/1 -> AEMS_DEM_TIMEBASEDDEBOUNCE/6

== system AEMS_Standard_Library/SUB/AEMS_DEM_TIME_BASED_DEBOUNCE_6D/AEMS_DEM_TIME_BASED_DEBOUNCE_CALL2 ==
  conditionfulfilled : Inport
  prefailed : Inport  Port=2
  prepassed : Inport  Port=3
  reseteventdebounce : Inport  Port=4
  DemDebounceBehavior : Inport  Port=5
  DemCounterFailedThreshold : Inport  Port=6
  DemCounterPassedThreshold : Inport  Port=7
  Enable : EnablePort
  AEMS_DEM_TIMEBASEDDEBOUNCE : AEMS_Standard_Library/SUB/AEMS_DEM_TIMEBASEDDEBOUNCE  Tag=[LIB]  eventid=Dem_EventId_Device2_Faulttype  sampletime=0.01
      settings: AttributesFormatString=|
      | %<MaskType>
      | EventId: %<eventid>
      | Sample time: %<sampletime>
  debouncevalue_for_failed : Outport
  debouncevalue_for_passed : Outport  Port=2
  failed : Outport  Port=3
  passed : Outport  Port=4
  wires:
  DemCounterPassedThreshold/1 -> AEMS_DEM_TIMEBASEDDEBOUNCE/6
  DemDebounceBehavior/1 -> AEMS_DEM_TIMEBASEDDEBOUNCE/4
  conditionfulfilled/1 -> AEMS_DEM_TIMEBASEDDEBOUNCE/1
  prepassed/1 -> AEMS_DEM_TIMEBASEDDEBOUNCE/3
  reseteventdebounce/1 -> AEMS_DEM_TIMEBASEDDEBOUNCE/7
  prefailed/1 -> AEMS_DEM_TIMEBASEDDEBOUNCE/2
  DemCounterFailedThreshold/1 -> AEMS_DEM_TIMEBASEDDEBOUNCE/5
  AEMS_DEM_TIMEBASEDDEBOUNCE/1 -> debouncevalue_for_failed/1
  AEMS_DEM_TIMEBASEDDEBOUNCE/2 -> debouncevalue_for_passed/1
  AEMS_DEM_TIMEBASEDDEBOUNCE/3 -> failed/1
  AEMS_DEM_TIMEBASEDDEBOUNCE/4 -> passed/1

== system AEMS_Standard_Library/SUB/AEMS_DEM_TIME_BASED_DEBOUNCE_6D/AEMS_DEM_TIME_BASED_DEBOUNCE_CALL3 ==
  conditionfulfilled : Inport
  prefailed : Inport  Port=2
  prepassed : Inport  Port=3
  reseteventdebounce : Inport  Port=4
  DemDebounceBehavior : Inport  Port=5
  DemCounterFailedThreshold : Inport  Port=6
  DemCounterPassedThreshold : Inport  Port=7
  Enable : EnablePort
  AEMS_DEM_TIMEBASEDDEBOUNCE : AEMS_Standard_Library/SUB/AEMS_DEM_TIMEBASEDDEBOUNCE  Tag=[LIB]  eventid=Dem_EventId_Device3_Faulttype  sampletime=0.01
      settings: AttributesFormatString=|
      | %<MaskType>
      | EventId: %<eventid>
      | Sample time: %<sampletime>
  debouncevalue_for_failed : Outport
  debouncevalue_for_passed : Outport  Port=2
  failed : Outport  Port=3
  passed : Outport  Port=4
  wires:
  DemCounterPassedThreshold/1 -> AEMS_DEM_TIMEBASEDDEBOUNCE/6
  DemDebounceBehavior/1 -> AEMS_DEM_TIMEBASEDDEBOUNCE/4
  conditionfulfilled/1 -> AEMS_DEM_TIMEBASEDDEBOUNCE/1
  prepassed/1 -> AEMS_DEM_TIMEBASEDDEBOUNCE/3
  reseteventdebounce/1 -> AEMS_DEM_TIMEBASEDDEBOUNCE/7
  prefailed/1 -> AEMS_DEM_TIMEBASEDDEBOUNCE/2
  DemCounterFailedThreshold/1 -> AEMS_DEM_TIMEBASEDDEBOUNCE/5
  AEMS_DEM_TIMEBASEDDEBOUNCE/1 -> debouncevalue_for_failed/1
  AEMS_DEM_TIMEBASEDDEBOUNCE/2 -> debouncevalue_for_passed/1
  AEMS_DEM_TIMEBASEDDEBOUNCE/3 -> failed/1
  AEMS_DEM_TIMEBASEDDEBOUNCE/4 -> passed/1

== system AEMS_Standard_Library/SUB/AEMS_DEM_TIME_BASED_DEBOUNCE_6D/AEMS_DEM_TIME_BASED_DEBOUNCE_CALL4 ==
  conditionfulfilled : Inport
  prefailed : Inport  Port=2
  prepassed : Inport  Port=3
  reseteventdebounce : Inport  Port=4
  DemDebounceBehavior : Inport  Port=5
  DemCounterFailedThreshold : Inport  Port=6
  DemCounterPassedThreshold : Inport  Port=7
  Enable : EnablePort
  AEMS_DEM_TIMEBASEDDEBOUNCE : AEMS_Standard_Library/SUB/AEMS_DEM_TIMEBASEDDEBOUNCE  Tag=[LIB]  eventid=Dem_EventId_Device4_Faulttype  sampletime=0.01
      settings: AttributesFormatString=|
      | %<MaskType>
      | EventId: %<eventid>
      | Sample time: %<sampletime>
  debouncevalue_for_failed : Outport
  debouncevalue_for_passed : Outport  Port=2
  failed : Outport  Port=3
  passed : Outport  Port=4
  wires:
  DemCounterPassedThreshold/1 -> AEMS_DEM_TIMEBASEDDEBOUNCE/6
  DemDebounceBehavior/1 -> AEMS_DEM_TIMEBASEDDEBOUNCE/4
  conditionfulfilled/1 -> AEMS_DEM_TIMEBASEDDEBOUNCE/1
  prepassed/1 -> AEMS_DEM_TIMEBASEDDEBOUNCE/3
  reseteventdebounce/1 -> AEMS_DEM_TIMEBASEDDEBOUNCE/7
  prefailed/1 -> AEMS_DEM_TIMEBASEDDEBOUNCE/2
  DemCounterFailedThreshold/1 -> AEMS_DEM_TIMEBASEDDEBOUNCE/5
  AEMS_DEM_TIMEBASEDDEBOUNCE/1 -> debouncevalue_for_failed/1
  AEMS_DEM_TIMEBASEDDEBOUNCE/2 -> debouncevalue_for_passed/1
  AEMS_DEM_TIMEBASEDDEBOUNCE/3 -> failed/1
  AEMS_DEM_TIMEBASEDDEBOUNCE/4 -> passed/1

== system AEMS_Standard_Library/SUB/AEMS_DEM_TIME_BASED_DEBOUNCE_6D/AEMS_DEM_TIME_BASED_DEBOUNCE_CALL5 ==
  conditionfulfilled : Inport
  prefailed : Inport  Port=2
  prepassed : Inport  Port=3
  reseteventdebounce : Inport  Port=4
  DemDebounceBehavior : Inport  Port=5
  DemCounterFailedThreshold : Inport  Port=6
  DemCounterPassedThreshold : Inport  Port=7
  Enable : EnablePort
  AEMS_DEM_TIMEBASEDDEBOUNCE : AEMS_Standard_Library/SUB/AEMS_DEM_TIMEBASEDDEBOUNCE  Tag=[LIB]  eventid=Dem_EventId_Device5_Faulttype  sampletime=0.01
      settings: AttributesFormatString=|
      | %<MaskType>
      | EventId: %<eventid>
      | Sample time: %<sampletime>
  debouncevalue_for_failed : Outport
  debouncevalue_for_passed : Outport  Port=2
  failed : Outport  Port=3
  passed : Outport  Port=4
  wires:
  DemCounterPassedThreshold/1 -> AEMS_DEM_TIMEBASEDDEBOUNCE/6
  DemDebounceBehavior/1 -> AEMS_DEM_TIMEBASEDDEBOUNCE/4
  conditionfulfilled/1 -> AEMS_DEM_TIMEBASEDDEBOUNCE/1
  prepassed/1 -> AEMS_DEM_TIMEBASEDDEBOUNCE/3
  reseteventdebounce/1 -> AEMS_DEM_TIMEBASEDDEBOUNCE/7
  prefailed/1 -> AEMS_DEM_TIMEBASEDDEBOUNCE/2
  DemCounterFailedThreshold/1 -> AEMS_DEM_TIMEBASEDDEBOUNCE/5
  AEMS_DEM_TIMEBASEDDEBOUNCE/1 -> debouncevalue_for_failed/1
  AEMS_DEM_TIMEBASEDDEBOUNCE/2 -> debouncevalue_for_passed/1
  AEMS_DEM_TIMEBASEDDEBOUNCE/3 -> failed/1
  AEMS_DEM_TIMEBASEDDEBOUNCE/4 -> passed/1

== system AEMS_Standard_Library/SUB/AEMS_DEM_TIME_BASED_DEBOUNCE_6D/AEMS_DEM_TIME_BASED_DEBOUNCE_CALL6 ==
  conditionfulfilled : Inport
  prefailed : Inport  Port=2
  prepassed : Inport  Port=3
  reseteventdebounce : Inport  Port=4
  DemDebounceBehavior : Inport  Port=5
  DemCounterFailedThreshold : Inport  Port=6
  DemCounterPassedThreshold : Inport  Port=7
  Enable : EnablePort
  AEMS_DEM_TIMEBASEDDEBOUNCE : AEMS_Standard_Library/SUB/AEMS_DEM_TIMEBASEDDEBOUNCE  Tag=[LIB]  eventid=Dem_EventId_Device6_Faulttype  sampletime=0.01
      settings: AttributesFormatString=|
      | %<MaskType>
      | EventId: %<eventid>
      | Sample time: %<sampletime>
  debouncevalue_for_failed : Outport
  debouncevalue_for_passed : Outport  Port=2
  failed : Outport  Port=3
  passed : Outport  Port=4
  wires:
  DemCounterPassedThreshold/1 -> AEMS_DEM_TIMEBASEDDEBOUNCE/6
  DemDebounceBehavior/1 -> AEMS_DEM_TIMEBASEDDEBOUNCE/4
  conditionfulfilled/1 -> AEMS_DEM_TIMEBASEDDEBOUNCE/1
  prepassed/1 -> AEMS_DEM_TIMEBASEDDEBOUNCE/3
  reseteventdebounce/1 -> AEMS_DEM_TIMEBASEDDEBOUNCE/7
  prefailed/1 -> AEMS_DEM_TIMEBASEDDEBOUNCE/2
  DemCounterFailedThreshold/1 -> AEMS_DEM_TIMEBASEDDEBOUNCE/5
  AEMS_DEM_TIMEBASEDDEBOUNCE/1 -> debouncevalue_for_failed/1
  AEMS_DEM_TIMEBASEDDEBOUNCE/2 -> debouncevalue_for_passed/1
  AEMS_DEM_TIMEBASEDDEBOUNCE/3 -> failed/1
  AEMS_DEM_TIMEBASEDDEBOUNCE/4 -> passed/1

== system AEMS_Standard_Library/SUB/AEMS_DEM_TIME_BASED_DEBOUNCE_8D/AEMS_DEM_TIME_BASED_DEBOUNCE_CALL1 ==
  conditionfulfilled : Inport
  prefailed : Inport  Port=2
  prepassed : Inport  Port=3
  reseteventdebounce : Inport  Port=4
  DemDebounceBehavior : Inport  Port=5
  DemCounterFailedThreshold : Inport  Port=6
  DemCounterPassedThreshold : Inport  Port=7
  Enable : EnablePort
  AEMS_DEM_TIMEBASEDDEBOUNCE : AEMS_Standard_Library/SUB/AEMS_DEM_TIMEBASEDDEBOUNCE  Tag=[LIB]  eventid=Dem_EventId_Device_Faulttype  sampletime=0.01
      settings: AttributesFormatString=|
      | %<MaskType>
      | EventId: %<eventid>
      | Sample time: %<sampletime>
  debouncevalue_for_failed : Outport
  debouncevalue_for_passed : Outport  Port=2
  failed : Outport  Port=3
  passed : Outport  Port=4
  wires:
  AEMS_DEM_TIMEBASEDDEBOUNCE/4 -> passed/1
  AEMS_DEM_TIMEBASEDDEBOUNCE/3 -> failed/1
  AEMS_DEM_TIMEBASEDDEBOUNCE/2 -> debouncevalue_for_passed/1
  AEMS_DEM_TIMEBASEDDEBOUNCE/1 -> debouncevalue_for_failed/1
  DemCounterFailedThreshold/1 -> AEMS_DEM_TIMEBASEDDEBOUNCE/5
  prefailed/1 -> AEMS_DEM_TIMEBASEDDEBOUNCE/2
  reseteventdebounce/1 -> AEMS_DEM_TIMEBASEDDEBOUNCE/7
  prepassed/1 -> AEMS_DEM_TIMEBASEDDEBOUNCE/3
  conditionfulfilled/1 -> AEMS_DEM_TIMEBASEDDEBOUNCE/1
  DemDebounceBehavior/1 -> AEMS_DEM_TIMEBASEDDEBOUNCE/4
  DemCounterPassedThreshold/1 -> AEMS_DEM_TIMEBASEDDEBOUNCE/6

== system AEMS_Standard_Library/SUB/AEMS_DEM_TIME_BASED_DEBOUNCE_8D/AEMS_DEM_TIME_BASED_DEBOUNCE_CALL2 ==
  conditionfulfilled : Inport
  prefailed : Inport  Port=2
  prepassed : Inport  Port=3
  reseteventdebounce : Inport  Port=4
  DemDebounceBehavior : Inport  Port=5
  DemCounterFailedThreshold : Inport  Port=6
  DemCounterPassedThreshold : Inport  Port=7
  Enable : EnablePort
  AEMS_DEM_TIMEBASEDDEBOUNCE : AEMS_Standard_Library/SUB/AEMS_DEM_TIMEBASEDDEBOUNCE  Tag=[LIB]  eventid=Dem_EventId_Device2_Faulttype  sampletime=0.01
      settings: AttributesFormatString=|
      | %<MaskType>
      | EventId: %<eventid>
      | Sample time: %<sampletime>
  debouncevalue_for_failed : Outport
  debouncevalue_for_passed : Outport  Port=2
  failed : Outport  Port=3
  passed : Outport  Port=4
  wires:
  DemCounterPassedThreshold/1 -> AEMS_DEM_TIMEBASEDDEBOUNCE/6
  DemDebounceBehavior/1 -> AEMS_DEM_TIMEBASEDDEBOUNCE/4
  conditionfulfilled/1 -> AEMS_DEM_TIMEBASEDDEBOUNCE/1
  prepassed/1 -> AEMS_DEM_TIMEBASEDDEBOUNCE/3
  reseteventdebounce/1 -> AEMS_DEM_TIMEBASEDDEBOUNCE/7
  prefailed/1 -> AEMS_DEM_TIMEBASEDDEBOUNCE/2
  DemCounterFailedThreshold/1 -> AEMS_DEM_TIMEBASEDDEBOUNCE/5
  AEMS_DEM_TIMEBASEDDEBOUNCE/1 -> debouncevalue_for_failed/1
  AEMS_DEM_TIMEBASEDDEBOUNCE/2 -> debouncevalue_for_passed/1
  AEMS_DEM_TIMEBASEDDEBOUNCE/3 -> failed/1
  AEMS_DEM_TIMEBASEDDEBOUNCE/4 -> passed/1

== system AEMS_Standard_Library/SUB/AEMS_DEM_TIME_BASED_DEBOUNCE_8D/AEMS_DEM_TIME_BASED_DEBOUNCE_CALL3 ==
  conditionfulfilled : Inport
  prefailed : Inport  Port=2
  prepassed : Inport  Port=3
  reseteventdebounce : Inport  Port=4
  DemDebounceBehavior : Inport  Port=5
  DemCounterFailedThreshold : Inport  Port=6
  DemCounterPassedThreshold : Inport  Port=7
  Enable : EnablePort
  AEMS_DEM_TIMEBASEDDEBOUNCE : AEMS_Standard_Library/SUB/AEMS_DEM_TIMEBASEDDEBOUNCE  Tag=[LIB]  eventid=Dem_EventId_Device3_Faulttype  sampletime=0.01
      settings: AttributesFormatString=|
      | %<MaskType>
      | EventId: %<eventid>
      | Sample time: %<sampletime>
  debouncevalue_for_failed : Outport
  debouncevalue_for_passed : Outport  Port=2
  failed : Outport  Port=3
  passed : Outport  Port=4
  wires:
  DemCounterPassedThreshold/1 -> AEMS_DEM_TIMEBASEDDEBOUNCE/6
  DemDebounceBehavior/1 -> AEMS_DEM_TIMEBASEDDEBOUNCE/4
  conditionfulfilled/1 -> AEMS_DEM_TIMEBASEDDEBOUNCE/1
  prepassed/1 -> AEMS_DEM_TIMEBASEDDEBOUNCE/3
  reseteventdebounce/1 -> AEMS_DEM_TIMEBASEDDEBOUNCE/7
  prefailed/1 -> AEMS_DEM_TIMEBASEDDEBOUNCE/2
  DemCounterFailedThreshold/1 -> AEMS_DEM_TIMEBASEDDEBOUNCE/5
  AEMS_DEM_TIMEBASEDDEBOUNCE/1 -> debouncevalue_for_failed/1
  AEMS_DEM_TIMEBASEDDEBOUNCE/2 -> debouncevalue_for_passed/1
  AEMS_DEM_TIMEBASEDDEBOUNCE/3 -> failed/1
  AEMS_DEM_TIMEBASEDDEBOUNCE/4 -> passed/1

== system AEMS_Standard_Library/SUB/AEMS_DEM_TIME_BASED_DEBOUNCE_8D/AEMS_DEM_TIME_BASED_DEBOUNCE_CALL4 ==
  conditionfulfilled : Inport
  prefailed : Inport  Port=2
  prepassed : Inport  Port=3
  reseteventdebounce : Inport  Port=4
  DemDebounceBehavior : Inport  Port=5
  DemCounterFailedThreshold : Inport  Port=6
  DemCounterPassedThreshold : Inport  Port=7
  Enable : EnablePort
  AEMS_DEM_TIMEBASEDDEBOUNCE : AEMS_Standard_Library/SUB/AEMS_DEM_TIMEBASEDDEBOUNCE  Tag=[LIB]  eventid=Dem_EventId_Device4_Faulttype  sampletime=0.01
      settings: AttributesFormatString=|
      | %<MaskType>
      | EventId: %<eventid>
      | Sample time: %<sampletime>
  debouncevalue_for_failed : Outport
  debouncevalue_for_passed : Outport  Port=2
  failed : Outport  Port=3
  passed : Outport  Port=4
  wires:
  DemCounterPassedThreshold/1 -> AEMS_DEM_TIMEBASEDDEBOUNCE/6
  DemDebounceBehavior/1 -> AEMS_DEM_TIMEBASEDDEBOUNCE/4
  conditionfulfilled/1 -> AEMS_DEM_TIMEBASEDDEBOUNCE/1
  prepassed/1 -> AEMS_DEM_TIMEBASEDDEBOUNCE/3
  reseteventdebounce/1 -> AEMS_DEM_TIMEBASEDDEBOUNCE/7
  prefailed/1 -> AEMS_DEM_TIMEBASEDDEBOUNCE/2
  DemCounterFailedThreshold/1 -> AEMS_DEM_TIMEBASEDDEBOUNCE/5
  AEMS_DEM_TIMEBASEDDEBOUNCE/1 -> debouncevalue_for_failed/1
  AEMS_DEM_TIMEBASEDDEBOUNCE/2 -> debouncevalue_for_passed/1
  AEMS_DEM_TIMEBASEDDEBOUNCE/3 -> failed/1
  AEMS_DEM_TIMEBASEDDEBOUNCE/4 -> passed/1

== system AEMS_Standard_Library/SUB/AEMS_DEM_TIME_BASED_DEBOUNCE_8D/AEMS_DEM_TIME_BASED_DEBOUNCE_CALL5 ==
  conditionfulfilled : Inport
  prefailed : Inport  Port=2
  prepassed : Inport  Port=3
  reseteventdebounce : Inport  Port=4
  DemDebounceBehavior : Inport  Port=5
  DemCounterFailedThreshold : Inport  Port=6
  DemCounterPassedThreshold : Inport  Port=7
  Enable : EnablePort
  AEMS_DEM_TIMEBASEDDEBOUNCE : AEMS_Standard_Library/SUB/AEMS_DEM_TIMEBASEDDEBOUNCE  Tag=[LIB]  eventid=Dem_EventId_Device5_Faulttype  sampletime=0.01
      settings: AttributesFormatString=|
      | %<MaskType>
      | EventId: %<eventid>
      | Sample time: %<sampletime>
  debouncevalue_for_failed : Outport
  debouncevalue_for_passed : Outport  Port=2
  failed : Outport  Port=3
  passed : Outport  Port=4
  wires:
  DemCounterPassedThreshold/1 -> AEMS_DEM_TIMEBASEDDEBOUNCE/6
  DemDebounceBehavior/1 -> AEMS_DEM_TIMEBASEDDEBOUNCE/4
  conditionfulfilled/1 -> AEMS_DEM_TIMEBASEDDEBOUNCE/1
  prepassed/1 -> AEMS_DEM_TIMEBASEDDEBOUNCE/3
  reseteventdebounce/1 -> AEMS_DEM_TIMEBASEDDEBOUNCE/7
  prefailed/1 -> AEMS_DEM_TIMEBASEDDEBOUNCE/2
  DemCounterFailedThreshold/1 -> AEMS_DEM_TIMEBASEDDEBOUNCE/5
  AEMS_DEM_TIMEBASEDDEBOUNCE/1 -> debouncevalue_for_failed/1
  AEMS_DEM_TIMEBASEDDEBOUNCE/2 -> debouncevalue_for_passed/1
  AEMS_DEM_TIMEBASEDDEBOUNCE/3 -> failed/1
  AEMS_DEM_TIMEBASEDDEBOUNCE/4 -> passed/1

== system AEMS_Standard_Library/SUB/AEMS_DEM_TIME_BASED_DEBOUNCE_8D/AEMS_DEM_TIME_BASED_DEBOUNCE_CALL6 ==
  conditionfulfilled : Inport
  prefailed : Inport  Port=2
  prepassed : Inport  Port=3
  reseteventdebounce : Inport  Port=4
  DemDebounceBehavior : Inport  Port=5
  DemCounterFailedThreshold : Inport  Port=6
  DemCounterPassedThreshold : Inport  Port=7
  Enable : EnablePort
  AEMS_DEM_TIMEBASEDDEBOUNCE : AEMS_Standard_Library/SUB/AEMS_DEM_TIMEBASEDDEBOUNCE  Tag=[LIB]  eventid=Dem_EventId_Device6_Faulttype  sampletime=0.01
      settings: AttributesFormatString=|
      | %<MaskType>
      | EventId: %<eventid>
      | Sample time: %<sampletime>
  debouncevalue_for_failed : Outport
  debouncevalue_for_passed : Outport  Port=2
  failed : Outport  Port=3
  passed : Outport  Port=4
  wires:
  DemCounterPassedThreshold/1 -> AEMS_DEM_TIMEBASEDDEBOUNCE/6
  DemDebounceBehavior/1 -> AEMS_DEM_TIMEBASEDDEBOUNCE/4
  conditionfulfilled/1 -> AEMS_DEM_TIMEBASEDDEBOUNCE/1
  prepassed/1 -> AEMS_DEM_TIMEBASEDDEBOUNCE/3
  reseteventdebounce/1 -> AEMS_DEM_TIMEBASEDDEBOUNCE/7
  prefailed/1 -> AEMS_DEM_TIMEBASEDDEBOUNCE/2
  DemCounterFailedThreshold/1 -> AEMS_DEM_TIMEBASEDDEBOUNCE/5
  AEMS_DEM_TIMEBASEDDEBOUNCE/1 -> debouncevalue_for_failed/1
  AEMS_DEM_TIMEBASEDDEBOUNCE/2 -> debouncevalue_for_passed/1
  AEMS_DEM_TIMEBASEDDEBOUNCE/3 -> failed/1
  AEMS_DEM_TIMEBASEDDEBOUNCE/4 -> passed/1

== system AEMS_Standard_Library/SUB/AEMS_DEM_TIME_BASED_DEBOUNCE_8D/AEMS_DEM_TIME_BASED_DEBOUNCE_CALL7 ==
  conditionfulfilled : Inport
  prefailed : Inport  Port=2
  prepassed : Inport  Port=3
  reseteventdebounce : Inport  Port=4
  DemDebounceBehavior : Inport  Port=5
  DemCounterFailedThreshold : Inport  Port=6
  DemCounterPassedThreshold : Inport  Port=7
  Enable : EnablePort
  AEMS_DEM_TIMEBASEDDEBOUNCE : AEMS_Standard_Library/SUB/AEMS_DEM_TIMEBASEDDEBOUNCE  Tag=[LIB]  eventid=Dem_EventId_Device7_Faulttype  sampletime=0.01
      settings: AttributesFormatString=|
      | %<MaskType>
      | EventId: %<eventid>
      | Sample time: %<sampletime>
  debouncevalue_for_failed : Outport
  debouncevalue_for_passed : Outport  Port=2
  failed : Outport  Port=3
  passed : Outport  Port=4
  wires:
  DemCounterPassedThreshold/1 -> AEMS_DEM_TIMEBASEDDEBOUNCE/6
  DemDebounceBehavior/1 -> AEMS_DEM_TIMEBASEDDEBOUNCE/4
  conditionfulfilled/1 -> AEMS_DEM_TIMEBASEDDEBOUNCE/1
  prepassed/1 -> AEMS_DEM_TIMEBASEDDEBOUNCE/3
  reseteventdebounce/1 -> AEMS_DEM_TIMEBASEDDEBOUNCE/7
  prefailed/1 -> AEMS_DEM_TIMEBASEDDEBOUNCE/2
  DemCounterFailedThreshold/1 -> AEMS_DEM_TIMEBASEDDEBOUNCE/5
  AEMS_DEM_TIMEBASEDDEBOUNCE/1 -> debouncevalue_for_failed/1
  AEMS_DEM_TIMEBASEDDEBOUNCE/2 -> debouncevalue_for_passed/1
  AEMS_DEM_TIMEBASEDDEBOUNCE/3 -> failed/1
  AEMS_DEM_TIMEBASEDDEBOUNCE/4 -> passed/1
